simulink model "Visualization"  (R2022b)
settings: Solver=FixedStepDiscrete  StartTime=0.0  StopTime=inf  FixedStep=0.001  RelTol=1e-3  EnableMultiTasking=on
undefined symbols (not defined in the file): localhost, qc_get_step_size
libraries: quarc_library x9
settings Model: SimulationMode=external  ExtModeTrigDuration=5000  Creator=glai  LastModifiedBy=lgonzalez
settings SolverCC: AlgebraicLoopSolver=TrustRegion  PositivePriorityOrder=on
settings DataIOCC: LimitDataPoints=on  SaveFormat=Array  ReturnWorkspaceOutputs=off
settings DebuggingCC: SolverPrmCheckMsg=warning  UnconnectedInputMsg=warning  UnconnectedOutputMsg=warning  UnconnectedLineMsg=warning  SFUnexpectedBacktrackingDiag=warning  SFNoUnconditionalDefaultTransitionDiag=warning  SFExecutionAtInitializationDiag=none  SFMachineParentedDataDiag=warning  ArithmeticOperatorsInVariantConditions=warning
settings ModelReferenceCC: EnableRefExpFcnMdlSchedulingChecks=on  PropagateSignalLabelsOutOfModel=off
settings SFSimCC: SimUseLocalCustomCode=off  CustomCodeUndefinedFunction=UseInterfaceOnly
settings RTWCC: Description=QUARC Win64 Target Using Toolchain  SystemTargetFile=quarc_win64.tlc  TemplateMakefile=quarc_default_tmf  RTWUseLocalCustomCode=off  Toolchain=QUARC win64 | nmake (64-bit Windows)  BuildConfiguration=Faster Runs
settings CodeAppCC: StateflowObjectComments=on
settings STFCustomTargetCC: ConcurrentExecutionCompliant=on  GRTInterface=on  UseToolchainInfoCompliant=on  SystemTargetFile=quarc_win64.tlc
settings GRTTargetCC: TargetLangStandard=C89/C90 (ANSI)  ParMdlRefBuildCompliant=off  CompOptLevelCompliant=off  CombineOutputUpdateFcns=off  MatFileLogging=off  CPPClassGenCompliant=off  GRTInterface=on  ExtMode=on  ExtModeMexFile=quarc_comm  ExtModeMexArgs='-w -d %d -uri %u', 'shmem://%m:1?timeout=10'
settings ConfigComp: CovMetricSettings=dw  CovSaveCumulativeToWorkspaceVar=on  CovSaveSingleToWorkspaceVar=on  CovExternalEMLEnable=off  CovSFcnEnable=off

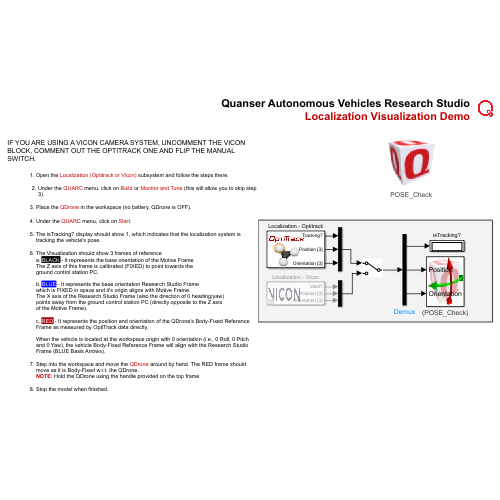
[thumbnail: Simulink's stored preview of the top-level diagram]
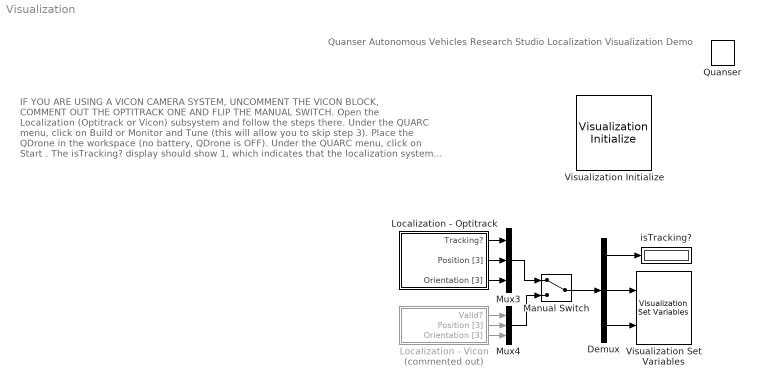
== system Visualization ==
  note: Quanser Autonomous Vehicles Research Studio
      | Localization Visualization Demo
  note: IF YOU ARE USING A VICON CAMERA SYSTEM, UNCOMMENT THE VICON BLOCK, COMMENT OUT THE OPTITRACK ONE AND FLIP THE MANUAL SWITCH.
      |
      | Open the Localization (Optitrack or Vicon) subsystem and follow the steps there.
      |
      | Under the QUARC menu, click on Build or Monitor and Tune (this will allow you to skip step 3).
      |
      | Place the QDrone in the workspace (no battery, QDrone is OFF).
      |
      | Under the QUARC menu, click on Start .
      |
      | The isTracking? display should show 1, which indicates that the localization system is tracking the vehicle's pose.
      |
      | The Visualization should show 3 frames of reference
      | a. BLACK - It represents the base orientation of the Motive Frame
      | The Z axis of this frame is calibrated (FIXED) to point towards the
      | ground control station PC.
      |
      | b. BLUE - It represents the base orientation Research Studio Frame
      | which is FIXED in space and it's origin aligns with Motive Frame.
      | The X axis of the Research Studio Frame (also the direction of 0 heading/yaw)
      | points away from the ground control station PC (directly opposite to the Z axis
      | of the Motive Frame).
      |
      | c. RED - It represents the position and orientation of the QDrone's Body-Fixed Reference Frame as measured by OptiTrack data directly.
      |
      | When the vehicle is located at the workspace origin with 0 orientation (i.e., 0 Roll, 0 Pitch and 0 Yaw), the vehicle Body-Fixed Reference Frame will align with the Research Studio Frame (BLUE Basis Arrows).
      |
      | Step into the workspace and move the QDrone around by hand. The RED frame should move as it is Body-Fixed w.r.t. the QDrone.
      | NOTE : Hold the QDrone using the handle provided on the top frame
      |
      | Stop the model when finished.
  Demux : Demux  Outputs=[1 3 3]
  Localization - Optitrack : Subsystem
      mask Display: image('optitrack.jpg')
  Localization - Vicon : Subsystem  Commented=on
      mask Display: image('vicon.jpg')
  Manual Switch : ManualSwitch
  Mux3 : Mux  Inputs=[1 3 3]
  Mux4 : Mux  Inputs=[1 3 3]
  Quanser : quarc_library/Logos/Quanser
  Visualization Initialize : quarc_library/User Interface/Visualization/Visualization Initialize  object_name=POSE_Check  scene_file=POSE_Check.xml  server_send_size=1000000  server_receive_size=1000  derive_from_server=on  client_send_size=1000  client_receive_size=1000000  variables=[ 60 61 ]  initial_values=single([ 0 0 0 0 0 0 ])  open_on_start=on  close_on_stop=on
      settings: AttributesFormatString=%<object_name>  SourceProductName=QUARC Targets
  Visualization Set Variables : quarc_library/User Interface/Visualization/Visualization Set Variables  object_name=POSE_Check  offset=[ 0 3 ]  data_type=[ 0 0 ]  length=[ 3 3 ]  sample_time=visualization_get_frame_period  actor_name={'actor.RefFrame.BodyFixed.OptiTrack/Position';'actor.RefFrame.BodyFixed.OptiTrack/Orientation'}
      settings: AttributesFormatString=(%<object_name>)  SourceProductName=QUARC Targets
  isTracking? : Display
  wires:
  Demux/2 -> Visualization Set Variables/1
  Demux/3 -> Visualization Set Variables/2
  Demux/1 -> isTracking?/1
  Localization - Optitrack/1(Tracking?) -> Mux3/1
  Localization - Optitrack/3(Orientation [3]) -> Mux3/3
  Mux3/1 -> Manual Switch/1
  Mux4/1 -> Manual Switch/2
  Localization - Vicon/2(Position [3]) -> Mux4/2
  Localization - Vicon/3(Orientation [3]) -> Mux4/3
  Localization - Vicon/1(Valid?) -> Mux4/1
  Localization - Optitrack/2(Position [3]) -> Mux3/2
  Manual Switch/1 -> Demux/1

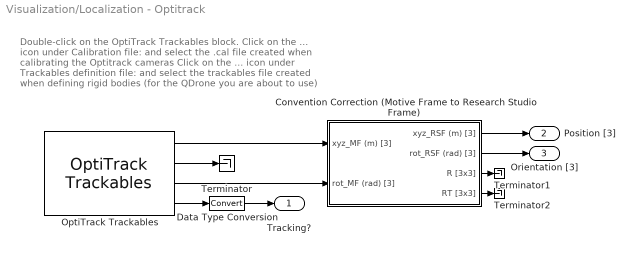
== system Visualization/Localization - Optitrack ==
  note: Double-click on the OptiTrack Trackables block.
      |
      | Click on the ... icon under Calibration file: and select the .cal file
      | created when calibrating the Optitrack cameras
      |
      | Click on the ... icon under Trackables definition file: and select
      | the trackables file created when defining rigid bodies (for the
      | QDrone you are about to use)
  Convention Correction (Motive Frame to Research Studio Frame) : Subsystem
  Data Type Conversion : DataTypeConversion  SaturateOnIntegerOverflow=off  RndMeth=Floor
  OptiTrack Trackables : quarc_library/Devices/Third-Party/NaturalPoint/OptiTrack/OptiTrack Trackables  calibration_file=C:\Users\user\Documents\OptiTrack\Session 2018-05-08\Calibration Exceptional (MeanErr 0.536 mm) 2018-05-08 10.cal  rigid_body_file=C:\Users\user\Documents\OptiTrack\Session 2018-05-08\Qdrone038682.tra  rigid_body_ids=[1]  sample_time=qc_get_step_size*10  active=off
      settings: SourceProductName=QUARC Targets
  Terminator : Terminator
  Terminator1 : Terminator
  Terminator2 : Terminator
  Tracking? : Outport  VectorParamsAs1DForOutWhenUnconnected=off
  Position [3] : Outport  Port=2  VectorParamsAs1DForOutWhenUnconnected=off
  Orientation [3] : Outport  Port=3  VectorParamsAs1DForOutWhenUnconnected=off
  wires:
  Convention Correction (Motive Frame to Research Studio Frame)/4(RT [3x3]) -> Terminator2/1
  OptiTrack Trackables/4 -> Data Type Conversion/1
  Data Type Conversion/1 -> Tracking?/1
  Convention Correction (Motive Frame to Research Studio Frame)/3(R [3x3]) -> Terminator1/1
  Convention Correction (Motive Frame to Research Studio Frame)/1(xyz_RSF (m) [3]) -> Position [3]/1
  OptiTrack Trackables/2 -> Terminator/1
  OptiTrack Trackables/3 -> Convention Correction (Motive Frame to Research Studio Frame)/2(rot_MF (rad) [3])
  OptiTrack Trackables/1 -> Convention Correction (Motive Frame to Research Studio Frame)/1(xyz_MF (m) [3])
  Convention Correction (Motive Frame to Research Studio Frame)/2(rot_RSF (rad) [3]) -> Orientation [3]/1

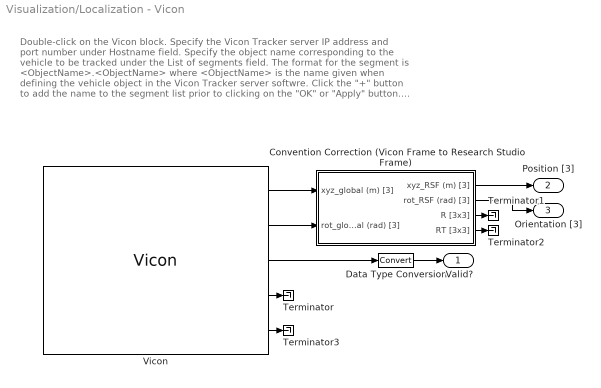
== system Visualization/Localization - Vicon ==
  note: Double-click on the Vicon block.
      |
      | Specify the Vicon Tracker server IP address and port number under Hostname field.
      |
      | Specify the object name corresponding to the vehicle to be tracked under the
      | List of segments field. The format for the segment is <ObjectName>.<ObjectName>
      | where <ObjectName> is the name given when defining the vehicle object in the
      | Vicon Tracker server softwre. Click the "+" button to add the name to the segment list
      | prior to clicking on the "OK" or "Apply" button.
      | Remove extra/unused entries from the list using the "-" button.
  Convention Correction (Vicon Frame to Research Studio Frame) : Subsystem
  Data Type Conversion : DataTypeConversion  SaturateOnIntegerOverflow=off  RndMeth=Floor
  Terminator{,1..3} (4 alike) : Terminator
  Vicon : quarc_library/Devices/Third-Party/Vicon/Vicon  hostname=localhost:801  segment_list=ObjectName1.ObjectName1\0\0  marker_list=\0  unlabeled_markers=[]  stream_mode=2  sample_time=qc_get_step_size  num_segments=1  num_markers=0  active=on
      settings: SourceProductName=QUARC Targets
  Valid? : Outport  VectorParamsAs1DForOutWhenUnconnected=off
  Position [3] : Outport  Port=2  VectorParamsAs1DForOutWhenUnconnected=off
  Orientation [3] : Outport  Port=3  VectorParamsAs1DForOutWhenUnconnected=off
  wires:
  Vicon/5 -> Terminator3/1
  Vicon/4 -> Terminator/1
  Convention Correction (Vicon Frame to Research Studio Frame)/1(xyz_RSF (m) [3]) -> Position [3]/1
  Convention Correction (Vicon Frame to Research Studio Frame)/4(RT [3x3]) -> Terminator2/1
  Vicon/3 -> Data Type Conversion/1
  Data Type Conversion/1 -> Valid?/1
  Convention Correction (Vicon Frame to Research Studio Frame)/2(rot_RSF (rad) [3]) -> Orientation [3]/1
  Vicon/2 -> Convention Correction (Vicon Frame to Research Studio Frame)/2(rot_global (rad) [3])
  Vicon/1 -> Convention Correction (Vicon Frame to Research Studio Frame)/1(xyz_global (m) [3])
  Convention Correction (Vicon Frame to Research Studio Frame)/3(R [3x3]) -> Terminator1/1

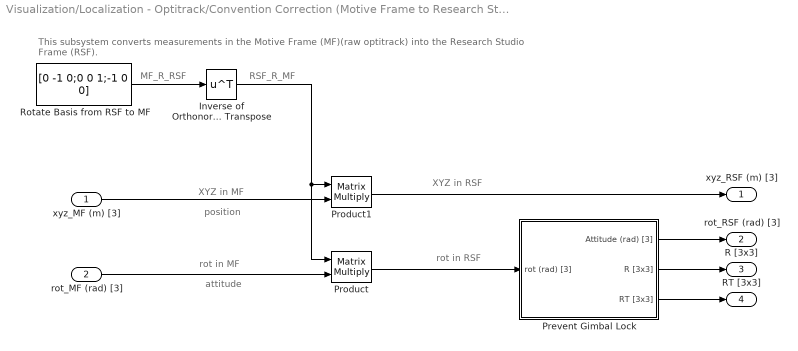
== system Visualization/Localization - Optitrack/Convention Correction (Motive Frame to Research Studio Frame) ==
  note: MF_R_RSF
  note: This subsystem converts measurements in the Motive Frame (MF)(raw optitrack) into the Research Studio Frame (RSF).
  note: RSF_R_MF
  note: XYZ in MF
  note: rot in MF
  note: position
  note: attitude
  note: XYZ in RSF
  note: rot in RSF
  xyz_MF (m) [3] : Inport
  rot_MF (rad) [3] : Inport  Port=2
  Inverse of Orthonormal Matrix is its Transpose : Math  Operator=transpose  SignedPower=on
  Prevent Gimbal Lock : Subsystem
  Product : Product  Multiplication=Matrix(*)
  Product1 : Product  Multiplication=Matrix(*)
  Rotate Basis from RSF to MF : Constant  Value=[0 -1 0;0 0 1;-1 0 0]
  xyz_RSF (m) [3] : Outport  VectorParamsAs1DForOutWhenUnconnected=off
  rot_RSF (rad) [3] : Outport  Port=2  VectorParamsAs1DForOutWhenUnconnected=off
  R [3x3] : Outport  Port=3  VectorParamsAs1DForOutWhenUnconnected=off
  RT [3x3] : Outport  Port=4  VectorParamsAs1DForOutWhenUnconnected=off
  wires:
  Rotate Basis from RSF to MF/1 -> Inverse of Orthonormal Matrix is its Transpose/1
  xyz_MF (m) [3]/1 -> Product1/2
  Inverse of Orthonormal Matrix is its Transpose/1 -> Product1/1, Product/1
  rot_MF (rad) [3]/1 -> Product/2
  Product1/1 -> xyz_RSF (m) [3]/1
  Product/1 -> Prevent Gimbal Lock/1(rot (rad) [3])
  Prevent Gimbal Lock/1(Attitude (rad) [3]) -> rot_RSF (rad) [3]/1
  Prevent Gimbal Lock/2(R [3x3]) -> R [3x3]/1
  Prevent Gimbal Lock/3(RT [3x3]) -> RT [3x3]/1

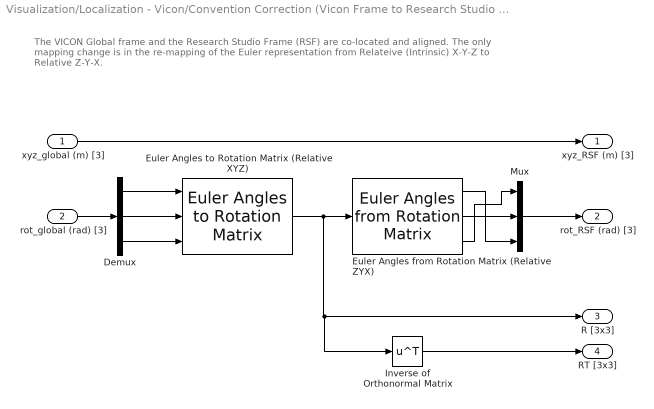
== system Visualization/Localization - Vicon/Convention Correction (Vicon Frame to Research Studio Frame) ==
  note: The VICON Global frame and the Research Studio Frame (RSF) are co-located and aligned.
      | The only mapping change is in the re-mapping of the Euler representation from
      | Relateive (Intrinsic) X-Y-Z to Relative Z-Y-X.
  xyz_global (m) [3] : Inport
  rot_global (rad) [3] : Inport  Port=2
  Demux : Demux  Outputs=3
  Euler Angles from Rotation Matrix (Relative ZYX) : quarc_library/Math Operations/Matrices/Euler Angles from Rotation Matrix  menu_order=Relative Z-Y-X
      settings: SourceProductName=QUARC Targets
  Euler Angles to Rotation Matrix (Relative XYZ) : quarc_library/Math Operations/Matrices/Euler Angles to Rotation Matrix  menu_order=Relative X-Y-Z
      settings: SourceProductName=QUARC Targets
  Inverse of Orthonormal Matrix : Math  Operator=transpose  SignedPower=on
  Mux : Mux  Inputs=3
  xyz_RSF (m) [3] : Outport  VectorParamsAs1DForOutWhenUnconnected=off
  rot_RSF (rad) [3] : Outport  Port=2  VectorParamsAs1DForOutWhenUnconnected=off
  R [3x3] : Outport  Port=3  VectorParamsAs1DForOutWhenUnconnected=off
  RT [3x3] : Outport  Port=4  VectorParamsAs1DForOutWhenUnconnected=off
  wires:
  Demux/3 -> Euler Angles to Rotation Matrix (Relative XYZ)/3
  Demux/1 -> Euler Angles to Rotation Matrix (Relative XYZ)/1
  rot_global (rad) [3]/1 -> Demux/1
  Demux/2 -> Euler Angles to Rotation Matrix (Relative XYZ)/2
  xyz_global (m) [3]/1 -> xyz_RSF (m) [3]/1
  Euler Angles from Rotation Matrix (Relative ZYX)/1 -> Mux/3
  Mux/1 -> rot_RSF (rad) [3]/1
  Euler Angles from Rotation Matrix (Relative ZYX)/3 -> Mux/1
  Euler Angles from Rotation Matrix (Relative ZYX)/2 -> Mux/2
  Euler Angles to Rotation Matrix (Relative XYZ)/1 -> Inverse of Orthonormal Matrix/1, R [3x3]/1, Euler Angles from Rotation Matrix (Relative ZYX)/1
  Inverse of Orthonormal Matrix/1 -> RT [3x3]/1

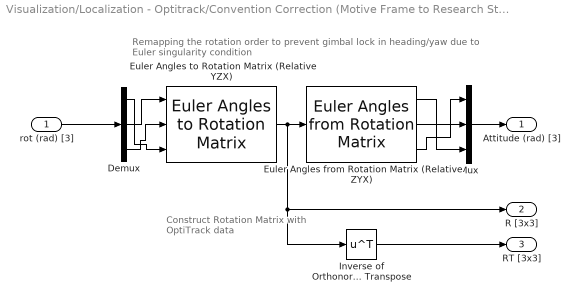
== system Visualization/Localization - Optitrack/Convention Correction (Motive Frame to Research Studio Frame)/Prevent Gimbal Lock ==
  note: Construct Rotation Matrix
      | with OptiTrack data
  note: Remapping the rotation order to prevent gimbal lock
      | in heading/yaw due to Euler singularity condition
  rot (rad) [3] : Inport
  Demux : Demux  Outputs=3
  Euler Angles from Rotation Matrix (Relative ZYX) : quarc_library/Math Operations/Matrices/Euler Angles from Rotation Matrix  menu_order=Relative Z-Y-X
      settings: SourceProductName=QUARC Targets
  Euler Angles to Rotation Matrix (Relative YZX) : quarc_library/Math Operations/Matrices/Euler Angles to Rotation Matrix  menu_order=Relative Y-Z-X
      settings: SourceProductName=QUARC Targets
  Inverse of Orthonormal Matrix is its Transpose : Math  Operator=transpose  SignedPower=on
  Mux : Mux  Inputs=3
  Attitude (rad) [3] : Outport  VectorParamsAs1DForOutWhenUnconnected=off
  R [3x3] : Outport  Port=2  VectorParamsAs1DForOutWhenUnconnected=off
  RT [3x3] : Outport  Port=3  VectorParamsAs1DForOutWhenUnconnected=off
  wires:
  Euler Angles from Rotation Matrix (Relative ZYX)/2 -> Mux/2
  Euler Angles from Rotation Matrix (Relative ZYX)/1 -> Mux/3
  Euler Angles from Rotation Matrix (Relative ZYX)/3 -> Mux/1
  Euler Angles to Rotation Matrix (Relative YZX)/1 -> R [3x3]/1, Inverse of Orthonormal Matrix is its Transpose/1, Euler Angles from Rotation Matrix (Relative ZYX)/1
  rot (rad) [3]/1 -> Demux/1
  Mux/1 -> Attitude (rad) [3]/1
  Demux/2 -> Euler Angles to Rotation Matrix (Relative YZX)/1
  Demux/3 -> Euler Angles to Rotation Matrix (Relative YZX)/2
  Demux/1 -> Euler Angles to Rotation Matrix (Relative YZX)/3
  Inverse of Orthonormal Matrix is its Transpose/1 -> RT [3x3]/1
